simulink model "pdl_linear_hw1"  (R2017a)
settings: Solver=VariableStepAuto  StartTime=0.0  StopTime=duration  RelTol=1e-3
values from neighbouring files (symbols this model uses):
  A = [0 0 1 0; 0 0 0 1; -k/M -m*g/M -b/M 0; k/(M*L) (m+M)*g/(M*L) b/(M*L) 0]    [pendulum_hw1.m]
  B = [0;0;1/M;-1/(M*L)]    [pendulum_hw1.m]
  E = [0 0;0 0;-1/M 0;1/(M*L) -1/(m*L)]    [pendulum_hw1.m]
  f_p = 0    [pendulum_hw1.m]
  Ts = 0.001    [pendulum_hw1.m]
  w_p = 0    [pendulum_hw1.m]
  X_0 = [0;1*pi/180;0;0]    [pendulum_hw1.m]
libraries: simulink x2
settings Model: Creator=Salmon  LastModifiedBy=Salmon

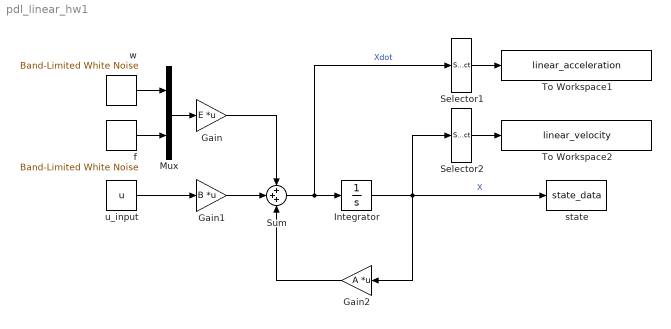
== system pdl_linear_hw1 ==
  Gain : Gain  Gain=E  Multiplication=Matrix(K*u)
  Gain1 : Gain  Gain=B  Multiplication=Matrix(K*u)
  Gain2 : Gain  Gain=A  Multiplication=Matrix(K*u)
  Integrator : Integrator  InitialCondition=X_0
  Mux : Mux  Inputs=2
  Selector1 : Selector  InputPortWidth=4  IndexOptions=Index vector (dialog)  Indices=[3]  OutputSizes=1
  Selector2 : Selector  InputPortWidth=4  IndexOptions=Index vector (dialog)  Indices=[3]  OutputSizes=1
  Sum : Sum  Inputs=+++
  To Workspace1 : ToWorkspace  VariableName=linear_acceleration  SaveFormat=Structure With Time  SampleTime=-1
  To Workspace2 : ToWorkspace  VariableName=linear_velocity  SaveFormat=Structure With Time  SampleTime=-1
  f : simulink/Sources/Band-Limited White Noise  Cov=[f_p]  Ts=Ts  seed=[23341]
  state : ToWorkspace  VariableName=state_data  SaveFormat=Structure With Time  SampleTime=Ts
  u_input : Constant  Value=u
  w : simulink/Sources/Band-Limited White Noise  Cov=[w_p]  Ts=Ts  seed=[23341]
  wires:
  w/1 -> Mux/1
  f/1 -> Mux/2
  Mux/1 -> Gain/1
  Gain1/1 -> Sum/2
  Sum/1 -> Integrator/1, Selector1/1  "Xdot"
  Gain2/1 -> Sum/3
  u_input/1 -> Gain1/1
  Gain/1 -> Sum/1
  Integrator/1 -> Gain2/1, Selector2/1, state/1  "X"
  Selector1/1 -> To Workspace1/1
  Selector2/1 -> To Workspace2/1
